simulink model "NewValidation"  (R2020b)
settings: Solver=VariableStepAuto  StartTime=0.0  StopTime=t_final  RelTol=1e-3
values from neighbouring files (symbols this model uses):
  A_eta = [zeros(3, 18) ... (first row only)    [NewSysIdentification.m]
  A_x = [zeros(3,3), eye(3,3),   zeros(3,3), zeros(3,1), zeros(3,3), zeros(3,1) ... (first row only)    [NewSysIdentification.m]
  B_u = [zeros(3,3) zeros(3,1) ... (first row only)    [NewSysIdentification.m]
  F_eta = H_DFL(dE + 1: dE + dG,      dX + 1: dX + dE     )    [NewSysIdentification.m]
  F_gamma = H_DFL(dE + 1: dE + dG, dX + dE + 1: dX + dE + dG)    [NewSysIdentification.m]
  F_u = H_DFL(dE + 1: dE + dG,dXi - dU + 1: dXi         )    [NewSysIdentification.m]
  F_x = H_DFL(dE + 1: dE + dG,           1: dX          )    [NewSysIdentification.m]
  H_eta = H_DFL(1:dE,      dX + 1: dX + dE     )    [NewSysIdentification.m]
  H_gamma = H_DFL(1:dE, dX + dE + 1: dX + dE + dG)    [NewSysIdentification.m]
  H_u = H_DFL(1:dE,dXi - dU + 1: dXi         )    [NewSysIdentification.m]
  H_x = H_DFL(1:dE,           1: dX          )    [NewSysIdentification.m]
  K = lqr(A,B,C_z'*Q_dfl*C_z,R)    [LQRCtrl.m]
  params = Parameters()    [GenerateTrainigInput.m]    (also in LQRCtrl.m = Parameters(th_0); NewGenerateTrainigInput.m = NewParameters(5 , 5); NewModelValidation.m = NewParameters(5, 5); NewSysIdentification.m = NewParameters)
settings Model: Creator=user  LastModifiedBy=sarmiento

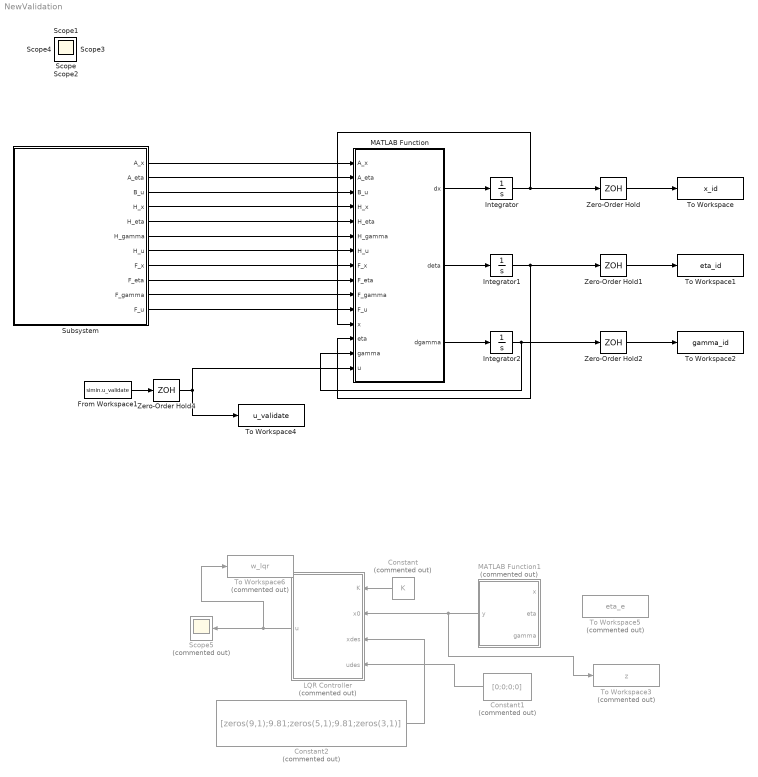
== system NewValidation ==
  Constant : Constant  Commented=on  Value=K
  Constant1 : Constant  Commented=on  Value=[0;0;0;0]
  Constant2 : Constant  Commented=on  Value=[zeros(9,1);9.81;zeros(5,1);9.81;zeros(3,1)]
  From Workspace1 : FromWorkspace  VariableName=simin.u_validate
  Integrator : Integrator  InitialCondition=params.x_0Taylor
  Integrator1 : Integrator  InitialCondition=params.eta_0
  Integrator2 : Integrator  InitialCondition=params.gamma_0
  LQR Controller : MATLAB Function  Commented=on  TreatAsAtomicUnit=on
  MATLAB Function : MATLAB Function  TreatAsAtomicUnit=on
  MATLAB Function1 : MATLAB Function  Commented=on  TreatAsAtomicUnit=on
  Scope5 : Scope  Commented=on
  Subsystem : Subsystem
  To Workspace : ToWorkspace  VariableName=x_id  SampleTime=-1
      settings: Save2DSignal=2-D array (concatenate along first dimension)
  To Workspace1 : ToWorkspace  VariableName=eta_id  SampleTime=-1
      settings: Save2DSignal=2-D array (concatenate along first dimension)
  To Workspace2 : ToWorkspace  VariableName=gamma_id  SampleTime=-1
      settings: Save2DSignal=2-D array (concatenate along first dimension)
  To Workspace3 : ToWorkspace  Commented=on  VariableName=z  SampleTime=-1
      settings: Save2DSignal=2-D array (concatenate along first dimension)
  To Workspace4 : ToWorkspace  VariableName=u_validate  SampleTime=-1
      settings: Save2DSignal=2-D array (concatenate along first dimension)
  To Workspace5 : ToWorkspace  Commented=on  VariableName=eta_e  SampleTime=-1
      settings: Save2DSignal=2-D array (concatenate along first dimension)
  To Workspace6 : ToWorkspace  Commented=on  VariableName=w_lqr  SampleTime=-1
      settings: Save2DSignal=2-D array (concatenate along first dimension)
  Zero-Order Hold{,1..2,4} (4 alike) : ZeroOrderHold  SampleTime=params.ST_id
  Scope{,1..4} (5 alike) : Scope
  wires:
  Subsystem/1(A_x) -> MATLAB Function/1(A_x)
  Subsystem/2(A_eta) -> MATLAB Function/2(A_eta)
  Subsystem/3(B_u) -> MATLAB Function/3(B_u)
  Subsystem/4(H_x) -> MATLAB Function/4(H_x)
  Subsystem/5(H_eta) -> MATLAB Function/5(H_eta)
  Subsystem/6(H_gamma) -> MATLAB Function/6(H_gamma)
  Subsystem/7(H_u) -> MATLAB Function/7(H_u)
  Subsystem/8(F_x) -> MATLAB Function/8(F_x)
  Subsystem/9(F_eta) -> MATLAB Function/9(F_eta)
  Subsystem/10(F_gamma) -> MATLAB Function/10(F_gamma)
  Subsystem/11(F_u) -> MATLAB Function/11(F_u)
  MATLAB Function/3(dgamma) -> Integrator2/1
  MATLAB Function/2(deta) -> Integrator1/1
  MATLAB Function/1(dx) -> Integrator/1
  Integrator/1 -> MATLAB Function/12(x), Zero-Order Hold/1
  Integrator1/1 -> Zero-Order Hold1/1, MATLAB Function/13(eta)
  Integrator2/1 -> Zero-Order Hold2/1, MATLAB Function/14(gamma)
  Zero-Order Hold/1 -> To Workspace/1
  Zero-Order Hold1/1 -> To Workspace1/1
  Zero-Order Hold2/1 -> To Workspace2/1
  Zero-Order Hold4/1 -> MATLAB Function/15(u), To Workspace4/1
  From Workspace1/1 -> Zero-Order Hold4/1
  MATLAB Function1/1(y) -> To Workspace3/1, LQR Controller/2(x0)
  Constant2/1 -> LQR Controller/3(xdes)
  Constant/1 -> LQR Controller/1(K)
  Constant1/1 -> LQR Controller/4(udes)
  LQR Controller/1(u) -> To Workspace6/1, Scope5/1

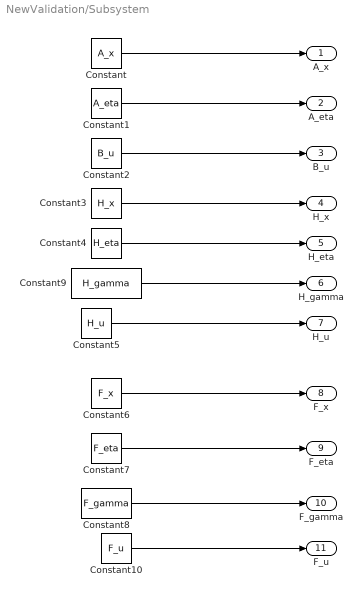
== system NewValidation/Subsystem ==
  Constant : Constant  Value=A_x
  Constant1 : Constant  Value=A_eta
  Constant10 : Constant  Value=F_u
  Constant2 : Constant  Value=B_u
  Constant3 : Constant  Value=H_x
  Constant4 : Constant  Value=H_eta
  Constant5 : Constant  Value=H_u
  Constant6 : Constant  Value=F_x
  Constant7 : Constant  Value=F_eta
  Constant8 : Constant  Value=F_gamma
  Constant9 : Constant  Value=H_gamma
  A_x : Outport
  A_eta : Outport  Port=2
  B_u : Outport  Port=3
  H_x : Outport  Port=4
  H_eta : Outport  Port=5
  H_gamma : Outport  Port=6
  H_u : Outport  Port=7
  F_x : Outport  Port=8
  F_eta : Outport  Port=9
  F_gamma : Outport  Port=10
  F_u : Outport  Port=11
  wires:
  Constant2/1 -> B_u/1
  Constant6/1 -> F_x/1
  Constant3/1 -> H_x/1
  Constant/1 -> A_x/1
  Constant4/1 -> H_eta/1
  Constant5/1 -> H_u/1
  Constant7/1 -> F_eta/1
  Constant8/1 -> F_gamma/1
  Constant10/1 -> F_u/1
  Constant1/1 -> A_eta/1
  Constant9/1 -> H_gamma/1

== matlab function NewValidation/MATLAB Function1 ==
  data: x input; y output; eta input; gamma input
function y = fcn(x,eta,gamma)

y = [x;eta;gamma];

== matlab function NewValidation/MATLAB Function ==
  data: A_x input; A_eta input; B_u input; H_x input; H_eta input; H_gamma input; H_u input; F_x input; F_eta input; F_gamma input; F_u input; x input; eta input; gamma input; u input; dx output; deta output; dgamma output
function [dx,deta,dgamma] = fcn(A_x,A_eta,B_u,H_x,H_eta,H_gamma,H_u,F_x,F_eta,F_gamma,F_u,x,eta,gamma,u)

A_gamma = zeros(14,size(gamma, 1));

dx = A_x*x + A_eta*eta + A_gamma*gamma + B_u*u;

deta = H_x*x + H_eta*eta + H_gamma*gamma + H_u*u;

dgamma = F_x*x + F_eta*eta + F_gamma*gamma + F_u*u;
% epsilon = x (7:9,:);
% eta_e = sqrt(1-epsilon'*epsilon);
end

== matlab function NewValidation/LQR Controller ==
  data: K input; u output; x0 input; xdes input; udes input
function u = fcn(K,x0,xdes,udes)
u = [0;0;0;0];
u = (udes - K*(x0-xdes));
